simulink model "narx_replay_validation"  (R2025b)
settings: Solver=FixedStepDiscrete  StartTime=0  StopTime=30000  FixedStep=1  RelTol=1e-3
libraries: neural x46
(part 2 of 2)

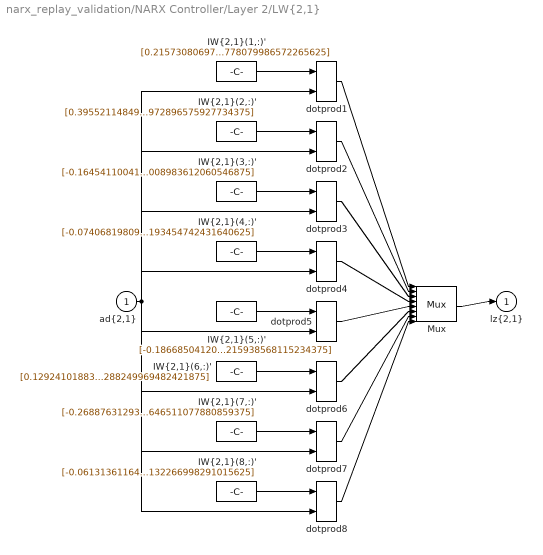
== system narx_replay_validation/NARX Controller/Layer 2/LW{2,1} ==
  "ad{2,1}" : Inport  PortDimensions=16  SampleTime=1
      mask Display: e = 0.06;c1 = [120 230 180]/255;c2 = ([120 230 180]+0)/(256+128);c3 = ([120 230 180]+128)/(256+128);patch([0 1 1 0],[0 0 1 1],c1);patch([0 1 1 1-e 1-e 0+e],[0 0 1 1-e 0+e 0+e],c2);patch([0 0 1 1-e 0+e 0+e],[0 1 1 1-e 1-e 0+e],c3);plot([0 1 1 0 0],[0 0 1 1 0]);
  "IW{2,1}(1,:)'" : Constant  Value=[0.215730806973578770335819854153669439256191253662109375;-0.031496284438560152862951468932806164957582950592041015625;-0.1395526553599035490815793991714599542319774627685546875;-0.04854907766490189346964001515516429208219051361083984375;-0.137535297754517171764376826104125939309597015380859375;-0.12115308480205556895814567042179987765848636627197265625;0.0847353869931739833720740762146306224167346954345703125;-0.235410614849904942236236138342064805328845977783203125;0.065990884543898176151088819096912629902362823486328125;-0.046756930354183760811803693968613515608012676239013671875;0.06787229889372110858136721844857675023376941680908203125;-0.1436465335325833037050102802822948433458805084228515625;-0.0135367264742757044404530830661315121687948703765869140625;-0.01179292928737141372963481700253396411426365375518798828125;0.1659868424309146328621267230118974111974239349365234375;0.0968118225912801000365703885108814574778079986572265625]
      mask Display: e = 0.06;c1 = [120 150 230]/255;c2 = ([120 150 230]+0)/383;c3 = ([120 150 230]+128)/383;patch([0 1 1 0],[0 0 1 1],c1);patch([0 1 1 1-e 1-e 0+e],[0 0 1 1-e 0+e 0+e],c2);patch([0 0 1 1-e 0+e 0+e],[0 1 1 1-e 1-e 0+e],c3);plot([0 1 1 0 0],[0 0 1 1 0]);disp('weights');
  "IW{2,1}(2,:)'" : Constant  Value=[0.39552114849365238580247705613146536052227020263671875;-0.1285454255295810366277464709128253161907196044921875;-0.2036144213910400235789666112395934760570526123046875;0.042260674794445292346001252781206858344376087188720703125;0.2013611641963235776575658064757590182125568389892578125;0.02744461059061804875103263157143373973667621612548828125;0.27157694500058748854343093626084737479686737060546875;-0.1489873447266756578688529089049552567303180694580078125;-0.162104742180245953164785532862879335880279541015625;-0.1387981496078161125495853411848656833171844482421875;0.1360147363599345238238669253405532799661159515380859375;-0.419585403435313419873153861772152595221996307373046875;-0.2494772641991747363920950419924338348209857940673828125;-0.06865373850929235022277907773968763649463653564453125;0.2302616585404423654726002723691635765135288238525390625;-0.01204159545533492990665447308629154576919972896575927734375]
      mask Display: e = 0.06;c1 = [120 150 230]/255;c2 = ([120 150 230]+0)/383;c3 = ([120 150 230]+128)/383;patch([0 1 1 0],[0 0 1 1],c1);patch([0 1 1 1-e 1-e 0+e],[0 0 1 1-e 0+e 0+e],c2);patch([0 0 1 1-e 0+e 0+e],[0 1 1 1-e 1-e 0+e],c3);plot([0 1 1 0 0],[0 0 1 1 0]);disp('weights');
  "IW{2,1}(3,:)'" : Constant  Value=[-0.1645411004134124388631477131639258004724979400634765625;0.09832055636181553925911913438540068455040454864501953125;0.0247172492236819203725861626708137919194996356964111328125;-0.1571521933237403911842733350567868910729885101318359375;-0.1066238943540271100207661447711871005594730377197265625;0.1341415701338838084577531617469503544270992279052734375;0.037141978756694470076293868032735190354287624359130859375;0.058893345238047623002586306029115803539752960205078125;0.04290146865315207225233251620011287741363048553466796875;-0.017641358155173557376027559939757338725030422210693359375;-0.040384946313995230549043213841287069953978061676025390625;0.049284838391954084724222440172525239177048206329345703125;0.0280503025257010270288038356056858901865780353546142578125;-0.0682246196915303471097757892493973486125469207763671875;-0.063512850463850634152862539849593304097652435302734375;0.09162321301618041313741258591107907705008983612060546875]
      mask Display: e = 0.06;c1 = [120 150 230]/255;c2 = ([120 150 230]+0)/383;c3 = ([120 150 230]+128)/383;patch([0 1 1 0],[0 0 1 1],c1);patch([0 1 1 1-e 1-e 0+e],[0 0 1 1-e 0+e 0+e],c2);patch([0 0 1 1-e 0+e 0+e],[0 1 1 1-e 1-e 0+e],c3);plot([0 1 1 0 0],[0 0 1 1 0]);disp('weights');
  "IW{2,1}(4,:)'" : Constant  Value=[-0.0740681980904032422063920648724888451397418975830078125;0.04984104822557706981900338405466754920780658721923828125;0.0656696601148659964142240141882211901247501373291015625;-0.0610309535264368374640753245330415666103363037109375;-0.051276607925690324829570698739189538173377513885498046875;0.07289241002515588208066077413604944013059139251708984375;-0.07326439948884823361030527166803949512541294097900390625;0.07904056529491811089460640005199820734560489654541015625;-0.033539231710676263575887645629336475394666194915771484375;0.0333477277518626491481512630343786440789699554443359375;0.044716296632350431561331305374551448039710521697998046875;0.11872255857273660006878657213746919296681880950927734375;0.0250931653597422886503576222594347200356423854827880859375;0.006968750033236039038986309179790623602457344532012939453125;-0.0384554596690623584631651965537457726895809173583984375;0.0503696638641125959967581593446084298193454742431640625]
      mask Display: e = 0.06;c1 = [120 150 230]/255;c2 = ([120 150 230]+0)/383;c3 = ([120 150 230]+128)/383;patch([0 1 1 0],[0 0 1 1],c1);patch([0 1 1 1-e 1-e 0+e],[0 0 1 1-e 0+e 0+e],c2);patch([0 0 1 1-e 0+e 0+e],[0 1 1 1-e 1-e 0+e],c3);plot([0 1 1 0 0],[0 0 1 1 0]);disp('weights');
  "IW{2,1}(5,:)'" : Constant  Value=[-0.1866850412065848008325019691255874931812286376953125;0.3188250694137757523805021264706738293170928955078125;-0.0059171961816270983447463294169210712425410747528076171875;-0.1446145290466320509903397351081366650760173797607421875;-0.25781727049642666482753838863573037087917327880859375;0.21946681267353207456238806116743944585323333740234375;0.06385585906620028229241370354429818689823150634765625;-0.10252012068670020294991473974732798524200916290283203125;0.12351706997365687057399696868742466904222965240478515625;-0.02536111008267437350038875365498824976384639739990234375;-0.1372883341959485192784740092974971048533916473388671875;0.178527549787153516636095673675299622118473052978515625;-0.007811364674959873910520258277756511233747005462646484375;-0.2044510863886282725498944046194083057343959808349609375;-0.1852864868100862205668732940466725267469882965087890625;-0.046266560842433933353756714268456562422215938568115234375]
      mask Display: e = 0.06;c1 = [120 150 230]/255;c2 = ([120 150 230]+0)/383;c3 = ([120 150 230]+128)/383;patch([0 1 1 0],[0 0 1 1],c1);patch([0 1 1 1-e 1-e 0+e],[0 0 1 1-e 0+e 0+e],c2);patch([0 0 1 1-e 0+e 0+e],[0 1 1 1-e 1-e 0+e],c3);plot([0 1 1 0 0],[0 0 1 1 0]);disp('weights');
  "IW{2,1}(6,:)'" : Constant  Value=[0.1292410188398716297530910424029571004211902618408203125;-0.22462180068346604411289035851950757205486297607421875;0.00858912054548042168400368012726175948046147823333740234375;0.588226218777996745501468467409722506999969482421875;0.3502857203712481659607647088705562055110931396484375;-0.245581606127061091715546581326634623110294342041015625;-0.260693475250822703781494737995672039687633514404296875;0.2039376711422458965383697204742929898202419281005859375;-0.260174844940660510150820527996984310448169708251953125;0.226716673592053219454811596733634360134601593017578125;-0.0105841120235892031942182001102992217056453227996826171875;-0.11732358797450055665212431676991400308907032012939453125;0.07334578676636417660095190740321413613855838775634765625;-0.1497033789901237310626669341218075715005397796630859375;0.136078440712464165951445238533779047429561614990234375;0.1308945729082422182454337189483339898288249969482421875]
      mask Display: e = 0.06;c1 = [120 150 230]/255;c2 = ([120 150 230]+0)/383;c3 = ([120 150 230]+128)/383;patch([0 1 1 0],[0 0 1 1],c1);patch([0 1 1 1-e 1-e 0+e],[0 0 1 1-e 0+e 0+e],c2);patch([0 0 1 1-e 0+e 0+e],[0 1 1 1-e 1-e 0+e],c3);plot([0 1 1 0 0],[0 0 1 1 0]);disp('weights');
  "IW{2,1}(7,:)'" : Constant  Value=[-0.268876312937278594272783038832130841910839080810546875;0.16297618733556806791540338963386602699756622314453125;0.143335466367658426189990450438926927745342254638671875;-0.1574722485266931981673366180984885431826114654541015625;-0.0960709442625411469407481490634381771087646484375;0.26464500053579786964519371394999325275421142578125;-0.0836951769327154149191727583456668071448802947998046875;0.06656448610722665026884214967139996588230133056640625;0.13892020088719159165435712566250003874301910400390625;-0.0595768044463832746604481371832662262022495269775390625;-0.007373864338918477423501229850444360636174678802490234375;0.00760489434531500148317650911167220328934490680694580078125;-0.00578747811459555394630882574347197078168392181396484375;-0.129202661535047891305794109939597547054290771484375;-0.264558194168394267276056552873342297971248626708984375;-0.039268489877851940617059511851039133034646511077880859375]
      mask Display: e = 0.06;c1 = [120 150 230]/255;c2 = ([120 150 230]+0)/383;c3 = ([120 150 230]+128)/383;patch([0 1 1 0],[0 0 1 1],c1);patch([0 1 1 1-e 1-e 0+e],[0 0 1 1-e 0+e 0+e],c2);patch([0 0 1 1-e 0+e 0+e],[0 1 1 1-e 1-e 0+e],c3);plot([0 1 1 0 0],[0 0 1 1 0]);disp('weights');
  "IW{2,1}(8,:)'" : Constant  Value=[-0.061313611642139963231468158255665912292897701263427734375;0.0155496894511459628207550309753059991635382175445556640625;0.0420811417152156252985406581501592881977558135986328125;-0.04344048406520183147616620544795296154916286468505859375;-0.0032844921325703379209881571654250365099869668483734130859375;0.043364171758223997443781883021074463613331317901611328125;-0.03168008455899740116734619732596911489963531494140625;-0.0214258816558940932972543436108026071451604366302490234375;0.03869448937403807686763457240886054933071136474609375;-0.033879764602411925611402665481364238075911998748779296875;0.024062972741498094009227060041666845791041851043701171875;-0.01556738716498822124034706604334132862277328968048095703125;-0.01604395875250634595499121815009857527911663055419921875;0.0107771176046396188752396483323536813259124755859375;-0.059166445181532349717468122207719716243445873260498046875;-0.00801442514058941547772096924973084242083132266998291015625]
      mask Display: e = 0.06;c1 = [120 150 230]/255;c2 = ([120 150 230]+0)/383;c3 = ([120 150 230]+128)/383;patch([0 1 1 0],[0 0 1 1],c1);patch([0 1 1 1-e 1-e 0+e],[0 0 1 1-e 0+e 0+e],c2);patch([0 0 1 1-e 0+e 0+e],[0 1 1 1-e 1-e 0+e],c3);plot([0 1 1 0 0],[0 0 1 1 0]);disp('weights');
  Mux : Mux  Inputs=8
      mask Display: e = 0.06;c1 = [120 150 230]/255;c2 = ([120 150 230]+0)/383;c3 = ([120 150 230]+128)/383;patch([0 1 1 0],[0 0 1 1],c1);patch([0 1 1 1-e 1-e 0+e],[0 0 1 1-e 0+e 0+e],c2);patch([0 0 1 1-e 0+e 0+e],[0 1 1 1-e 1-e 0+e],c3);plot([0 1 1 0 0],[0 0 1 1 0]);disp('Mux');
  dotprod{1..8} (8 alike) : neural/Weight Functions/dotprod
  "lz{2,1}" : Outport
      mask Display: e = 0.06;c1 = [120 230 180]/255;c2 = ([120 230 180]+0)/(256+128);c3 = ([120 230 180]+128)/(256+128);patch([0 1 1 0],[0 0 1 1],c1);patch([0 1 1 1-e 1-e 0+e],[0 0 1 1-e 0+e 0+e],c2);patch([0 0 1 1-e 0+e 0+e],[0 1 1 1-e 1-e 0+e],c3);plot([0 1 1 0 0],[0 0 1 1 0]);
  wires:
  "IW{2,1}(1,:)'"/1 -> dotprod1/1
  "ad{2,1}"/1 -> dotprod1/2, dotprod2/2, dotprod3/2, dotprod4/2, dotprod5/2, dotprod6/2, dotprod7/2, dotprod8/2
  dotprod1/1 -> Mux/1
  "IW{2,1}(2,:)'"/1 -> dotprod2/1
  dotprod2/1 -> Mux/2
  "IW{2,1}(3,:)'"/1 -> dotprod3/1
  dotprod3/1 -> Mux/3
  "IW{2,1}(4,:)'"/1 -> dotprod4/1
  dotprod4/1 -> Mux/4
  "IW{2,1}(5,:)'"/1 -> dotprod5/1
  dotprod5/1 -> Mux/5
  "IW{2,1}(6,:)'"/1 -> dotprod6/1
  dotprod6/1 -> Mux/6
  "IW{2,1}(7,:)'"/1 -> dotprod7/1
  dotprod7/1 -> Mux/7
  "IW{2,1}(8,:)'"/1 -> dotprod8/1
  dotprod8/1 -> Mux/8
  Mux/1 -> "lz{2,1}"/1

== system narx_replay_validation/NARX Controller/Layer 3/Delays 1 ==
  "p{3}" : Inport  PortDimensions=8  SampleTime=1
      mask Display: e = 0.06;c1 = [120 230 180]/255;c2 = ([120 230 180]+0)/(256+128);c3 = ([120 230 180]+128)/(256+128);patch([0 1 1 0],[0 0 1 1],c1);patch([0 1 1 1-e 1-e 0+e],[0 0 1 1-e 0+e 0+e],c2);patch([0 0 1 1-e 0+e 0+e],[0 1 1 1-e 1-e 0+e],c3);plot([0 1 1 0 0],[0 0 1 1 0]);
  mux : Mux  Inputs=1
      mask Display: e = 0.06;c1 = [120 150 230]/255;c2 = ([120 150 230]+0)/383;c3 = ([120 150 230]+128)/383;patch([0 1 1 0],[0 0 1 1],c1);patch([0 1 1 1-e 1-e 0+e],[0 0 1 1-e 0+e 0+e],c2);patch([0 0 1 1-e 0+e 0+e],[0 1 1 1-e 1-e 0+e],c3);plot([0 1 1 0 0],[0 0 1 1 0]);disp('Mux')
  "pd{3,2}" : Outport
      mask Display: e = 0.06;c1 = [120 230 180]/255;c2 = ([120 230 180]+0)/(256+128);c3 = ([120 230 180]+128)/(256+128);patch([0 1 1 0],[0 0 1 1],c1);patch([0 1 1 1-e 1-e 0+e],[0 0 1 1-e 0+e 0+e],c2);patch([0 0 1 1-e 0+e 0+e],[0 1 1 1-e 1-e 0+e],c3);plot([0 1 1 0 0],[0 0 1 1 0]);
  wires:
  "p{3}"/1 -> mux/1
  mux/1 -> "pd{3,2}"/1

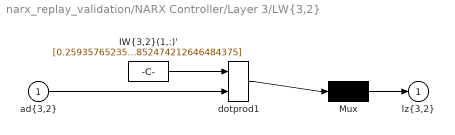
== system narx_replay_validation/NARX Controller/Layer 3/LW{3,2} ==
  "ad{3,2}" : Inport  PortDimensions=8  SampleTime=1
      mask Display: e = 0.06;c1 = [120 230 180]/255;c2 = ([120 230 180]+0)/(256+128);c3 = ([120 230 180]+128)/(256+128);patch([0 1 1 0],[0 0 1 1],c1);patch([0 1 1 1-e 1-e 0+e],[0 0 1 1-e 0+e 0+e],c2);patch([0 0 1 1-e 0+e 0+e],[0 1 1 1-e 1-e 0+e],c3);plot([0 1 1 0 0],[0 0 1 1 0]);
  "IW{3,2}(1,:)'" : Constant  Value=[0.259357652352828649267024729851982556283473968505859375;0.76634151003189832085382704462972469627857208251953125;0.02481443737775985980409387821055133827030658721923828125;-0.21141035778461925165316870334208942949771881103515625;-0.40328427339842443100081936790957115590572357177734375;0.75317540593005960491979067228385247290134429931640625;-0.373287135192127472738121696238522417843341827392578125;-0.11588875449453338306593508377773105166852474212646484375]
      mask Display: e = 0.06;c1 = [120 150 230]/255;c2 = ([120 150 230]+0)/383;c3 = ([120 150 230]+128)/383;patch([0 1 1 0],[0 0 1 1],c1);patch([0 1 1 1-e 1-e 0+e],[0 0 1 1-e 0+e 0+e],c2);patch([0 0 1 1-e 0+e 0+e],[0 1 1 1-e 1-e 0+e],c3);plot([0 1 1 0 0],[0 0 1 1 0]);disp('weights');
  Mux : Mux  Inputs=1
      mask Display: e = 0.06;c1 = [120 150 230]/255;c2 = ([120 150 230]+0)/383;c3 = ([120 150 230]+128)/383;patch([0 1 1 0],[0 0 1 1],c1);patch([0 1 1 1-e 1-e 0+e],[0 0 1 1-e 0+e 0+e],c2);patch([0 0 1 1-e 0+e 0+e],[0 1 1 1-e 1-e 0+e],c3);plot([0 1 1 0 0],[0 0 1 1 0]);disp('Mux');
  dotprod1 : neural/Weight Functions/dotprod
  "lz{3,2}" : Outport
      mask Display: e = 0.06;c1 = [120 230 180]/255;c2 = ([120 230 180]+0)/(256+128);c3 = ([120 230 180]+128)/(256+128);patch([0 1 1 0],[0 0 1 1],c1);patch([0 1 1 1-e 1-e 0+e],[0 0 1 1-e 0+e 0+e],c2);patch([0 0 1 1-e 0+e 0+e],[0 1 1 1-e 1-e 0+e],c3);plot([0 1 1 0 0],[0 0 1 1 0]);
  wires:
  "IW{3,2}(1,:)'"/1 -> dotprod1/1
  "ad{3,2}"/1 -> dotprod1/2
  dotprod1/1 -> Mux/1
  Mux/1 -> "lz{3,2}"/1
